simulink model "SISTEMA2"  (R2025b)
settings: Solver=ode23t  StartTime=0.0  StopTime=10.0  RelTol=1e-3
libraries: slpidlib x1, simulink x1
settings DataIOCC: ReturnWorkspaceOutputs=off  TimeSaveName=t
settings DebuggingCC: AlgebraicLoopMsg=none  ArtificialAlgebraicLoopMsg=none  MaxConsecutiveZCsMsg=none

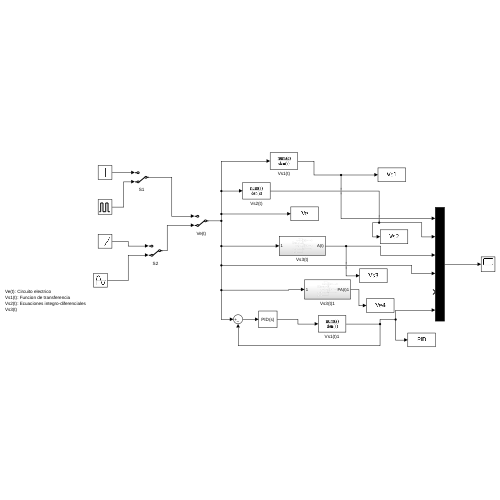
[thumbnail: Simulink's stored preview of the top-level diagram]
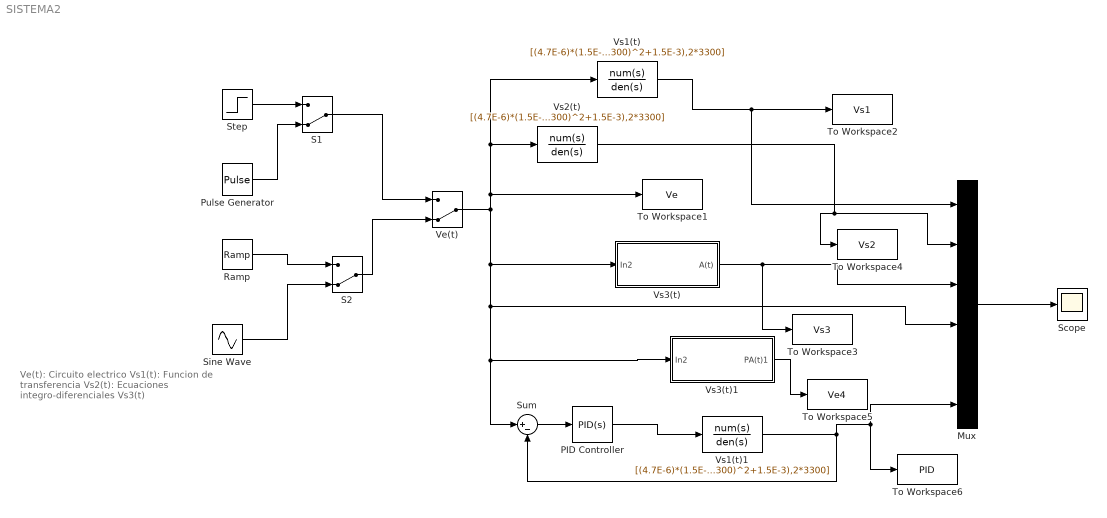
== system SISTEMA2 ==
  note: Ve(t): Circuito electrico
      | Vs1(t): Funcion de transferencia
      | Vs2(t): Ecuaciones integro-diferenciales
      | Vs3(t)
  Mux : Mux  Inputs=6
  PID Controller : slpidlib/PID Controller  Controller=PID  Form=Parallel  TimeDomain=Continuous-time  UseExternalTs=off  SampleTime=-1  IntegratorMethod=Forward Euler  FilterMethod=Forward Euler  ControllerParametersSource=internal  P=0  I=5826.83507312895  UseKiTs=off  D=0  UseExternalDerivativeSource=off  N=100  UseFilter=on  TunerSelectOption=Transfer Function Based (PID Tuner App)  InitialConditionSource=internal  InitialConditionForIntegrator=0  InitialConditionForFilter=0  DifferentiatorICPrevScaledInput=0  ExternalReset=none  TrackingMode=off  Kt=1  LimitOutput=off  SatLimitsSource=internal  UpperSaturationLimit=inf  LowerSaturationLimit=-inf  LinearizeAsGain=on  AntiWindupMode=none  Kb=1  LimitIntegrator=off  UpperIntegratorSaturationLimit=inf  LowerIntegratorSaturationLimit=-inf  POutMin=[]  POutMax=[]  IOutMin=[]  IOutMax=[]  DOutMin=[]  DOutMax=[]  NOutMin=[]  NOutMax=[]  SumOutMin=[]  SumOutMax=[]  SaturationOutMin=[]  SaturationOutMax=[]  PParamMin=[]  PParamMax=[]  IParamMin=[]  IParamMax=[]  DParamMin=[]  DParamMax=[]  NParamMin=[]  NParamMax=[]  KbParamMin=[]  KbParamMax=[]  KtParamMin=[]  KtParamMax=[]  KbOutMin=[]  KbOutMax=[]  KtOutMin=[]  KtOutMax=[]  IntegratorOutMin=[]  IntegratorOutMax=[]  FilterOutMin=[]  FilterOutMax=[]  SumI1OutMin=[]  SumI1OutMax=[]  SumI2OutMin=[]  SumI2OutMax=[]  SumI3OutMin=[]  SumI3OutMax=[]  SumI4OutMin=[]  SumI4OutMax=[]  SumDOutMin=[]  SumDOutMax=[]  DifferentiatorOutMin=[]  DifferentiatorOutMax=[]  FilterDiffOutCoefMin=[]  FilterDiffOutCoefMax=[]  ReciprocalOutMin=[]  ReciprocalOutMax=[]  SumDenOutMin=[]  SumDenOutMax=[]  SumNumOutMin=[]  SumNumOutMax=[]  DivideOutMin=[]  DivideOutMax=[]  UdiffTsProdOutMin=[]  UdiffTsProdOutMax=[]  NTsProdOutMin=[]  NTsProdOutMax=[]  UintegralTsProdOutMin=[]  UintegralTsProdOutMax=[]  UngainTsProdOutMin=[]  UngainTsProdOutMax=[]  ClampingZeroOutDataTypeStr=Inherit: Inherit via back propagation  ClampingZeroOutMin=[]  ClampingZeroOutMax=[]  FilterDenConstantOutDataTypeStr=Inherit: Inherit via back propagation  FilterDenConstantOutMin=[]  FilterDenConstantOutMax=[]  PCopyOutDataTypeStr=Inherit: Inherit via back propagation  PCopyOutMin=[]  PCopyOutMax=[]  NCopyOutDataTypeStr=Inherit: Inherit via back propagation  NCopyOutMin=[]  NCopyOutMax=[]  IntegratorContinuousStateAttributes=''  IntegratorStateMustResolveToSignalObject=off  IntegratorRTWStateStorageClass=Auto  FilterContinuousStateAttributes=''  FilterStateMustResolveToSignalObject=off  FilterRTWStateStorageClass=Auto  ParallelPVariant=InternalParameters  IdealPVariant=Disabled  IVariant=InternalParameters  DVariant=InternalParameters  IntegratorVariant=Continuous  SatVariant=Disabled  AWVariant=Passthrough  PCopyVariant=Disabled  TRVariant=Disabled  FdbkBlocksVariant=Forward  IdealPFdbkVariant=Disabled  SatFdbkVariant=Disabled  DerivativeFilterVariant=ContFilter  NVariant=InternalParameters  NCopyVariant=Disabled  FilterICVariant=InternalICsFilter  IntegratorICVariant=InternalICs  ExternalResetVariant=Disabled  TRSumVariant=Passthrough  SumFdbkVariant=Disabled  SumVariant=Sum_PID  TsampFilterVariant=InternalTs  TsampNgainVariant=Passthrough  TsampIntegralVariant=Disabled_SignalSpec  ExternalSaturationOutDataTypeStr=Inherit: Same as second input  DerivativeSourceVariant=ErrorSignal  PreIntVariant=InternalPreInt
  Pulse Generator : DiscretePulseGenerator  PulseType=Time based  Period=10  PulseWidth=10  PhaseDelay=1
  Ramp : simulink/Sources/Ramp  slope=1/10  start=0  InitialOutput=0
  S1 : ManualSwitch  CurrentSetting=0
  S2 : ManualSwitch  CurrentSetting=0
  Scope : Scope
      settings: ActiveDisplayYMinimum=-0.4451896203103759  ActiveDisplayYMaximum=1.4016296844259537
  Sine Wave : Sin  Frequency=pi/2  SampleTime=0
  Step : Step  Time=0  Before=1  SampleTime=0
  Sum : Sum  Inputs=|+-
  To Workspace1 : ToWorkspace  VariableName=Ve  SampleTime=-1
  To Workspace2 : ToWorkspace  VariableName=Vs1  SampleTime=-1
  To Workspace3 : ToWorkspace  VariableName=Vs3  SampleTime=-1
  To Workspace4 : ToWorkspace  VariableName=Vs2  SampleTime=-1
  To Workspace5 : ToWorkspace  VariableName=Ve4  SampleTime=-1
  To Workspace6 : ToWorkspace  VariableName=PID  SampleTime=-1
  Ve(t) : ManualSwitch  CurrentSetting=0
  Vs1(t) : TransferFcn  Numerator=[(4.7E-6)*(1.5E-3)*(3300),((4.7E-6)*(3300)^2+1.5E-3),3300]  Denominator=[3*(4.7E-6)*(1.5E-3)*3300,(5*(4.7E-6)*(3300)^2+1.5E-3),2*3300]
  Vs1(t)1 : TransferFcn  Numerator=[(4.7E-6)*(1.5E-3)*(3300),((4.7E-6)*(3300)^2+1.5E-3),3300]  Denominator=[3*(4.7E-6)*(1.5E-3)*3300,(5*(4.7E-6)*(3300)^2+1.5E-3),2*3300]
  Vs2(t) : TransferFcn  Numerator=[(4.7E-6)*(1.5E-3)*(3300),((4.7E-6)*(3300)^2+1.5E-3),3300]  Denominator=[3*(4.7E-6)*(1.5E-3)*3300,(5*(4.7E-6)*(3300)^2+1.5E-3),2*3300]
  Vs3(t) : Subsystem
  Vs3(t)1 : Subsystem
  wires:
  Step/1 -> S1/1
  Pulse Generator/1 -> S1/2
  Ramp/1 -> S2/1
  Sine Wave/1 -> S2/2
  S1/1 -> Ve(t)/1
  S2/1 -> Ve(t)/2
  Ve(t)/1 -> Vs3(t)/1(In2), Vs3(t)1/1(In2), Sum/1, Mux/4, Vs1(t)/1, Vs2(t)/1, To Workspace1/1
  Vs2(t)/1 -> Mux/2, To Workspace4/1
  Vs3(t)/1(A(t)) -> To Workspace3/1, Mux/3
  Mux/1 -> Scope/1
  Vs1(t)/1 -> To Workspace2/1, Mux/1
  Sum/1 -> PID Controller/1
  PID Controller/1 -> Vs1(t)1/1
  Vs1(t)1/1 -> Mux/6, To Workspace6/1, Sum/2
  Vs3(t)1/1(PA(t)1) -> To Workspace5/1

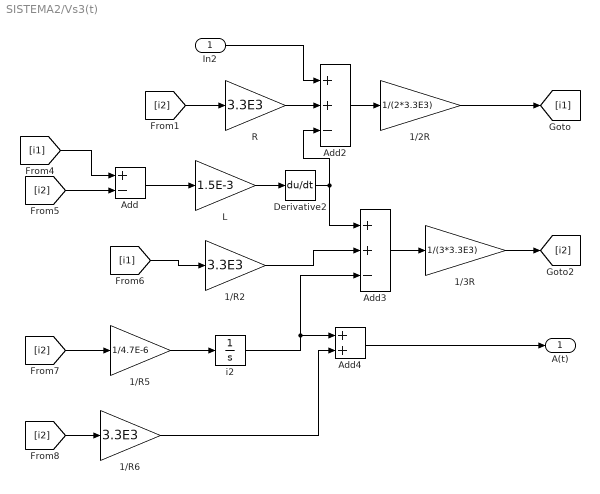
== system SISTEMA2/Vs3(t) ==
  In2 : Inport
  1/2R : Gain  Gain=1/(2*3.3E3)
  1/3R : Gain  Gain=1/(3*3.3E3)
  1/R2 : Gain  Gain=3.3E3
  1/R5 : Gain  Gain=1/4.7E-6
  1/R6 : Gain  Gain=3.3E3
  Add : Sum  Inputs=+-
  Add2 : Sum  Inputs=++-
  Add3 : Sum  Inputs=++-
  Add4 : Sum
  Derivative2 : Derivative
  L : Gain  Gain=1.5E-3
  R : Gain  Gain=3.3E3
  i2 : Integrator
  A(t) : Outport
  wires:
  1/2R/1 -> [i1]
  Add2/1 -> 1/2R/1
  In2/1 -> Add2/1
  [i2] -> R/1
  Derivative2/1 -> Add3/1, Add2/3
  L/1 -> Derivative2/1
  [i1] -> Add/1
  [i1] -> 1/R2/1
  1/R5/1 -> i2/1
  [i2] -> 1/R5/1
  R/1 -> Add2/2
  [i2] -> Add/2
  Add/1 -> L/1
  1/R2/1 -> Add3/2
  Add4/1 -> A(t)/1
  Add3/1 -> 1/3R/1
  1/3R/1 -> [i2]
  i2/1 -> Add4/1, Add3/3
  [i2] -> 1/R6/1
  1/R6/1 -> Add4/2

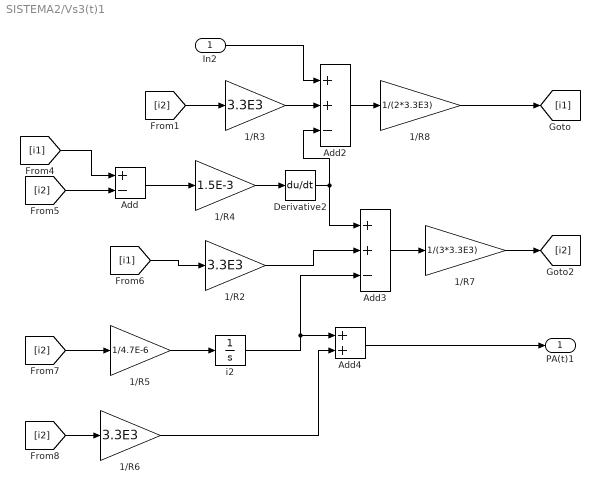
== system SISTEMA2/Vs3(t)1 ==
  In2 : Inport
  1/R2 : Gain  Gain=3.3E3
  1/R3 : Gain  Gain=3.3E3
  1/R4 : Gain  Gain=1.5E-3
  1/R5 : Gain  Gain=1/4.7E-6
  1/R6 : Gain  Gain=3.3E3
  1/R7 : Gain  Gain=1/(3*3.3E3)
  1/R8 : Gain  Gain=1/(2*3.3E3)
  Add : Sum  Inputs=+-
  Add2 : Sum  Inputs=++-
  Add3 : Sum  Inputs=++-
  Add4 : Sum
  Derivative2 : Derivative
  i2 : Integrator
  PA(t)1 : Outport
  wires:
  1/R8/1 -> [i1]
  Add2/1 -> 1/R8/1
  In2/1 -> Add2/1
  [i2] -> 1/R3/1
  Derivative2/1 -> Add3/1, Add2/3
  1/R4/1 -> Derivative2/1
  [i1] -> Add/1
  [i1] -> 1/R2/1
  1/R5/1 -> i2/1
  [i2] -> 1/R5/1
  1/R3/1 -> Add2/2
  [i2] -> Add/2
  Add/1 -> 1/R4/1
  1/R2/1 -> Add3/2
  Add4/1 -> PA(t)1/1
  Add3/1 -> 1/R7/1
  1/R7/1 -> [i2]
  i2/1 -> Add4/1, Add3/3
  [i2] -> 1/R6/1
  1/R6/1 -> Add4/2
